simulink subsystem "Sensor"  (R2023b)
settings: Solver=VariableStepAuto  StartTime=0.0  StopTime=10.0  RelTol=1e-3
libraries: arduinosensorlib x2
settings Model: Creator=Usuario_UMA  LastModifiedBy=Diego

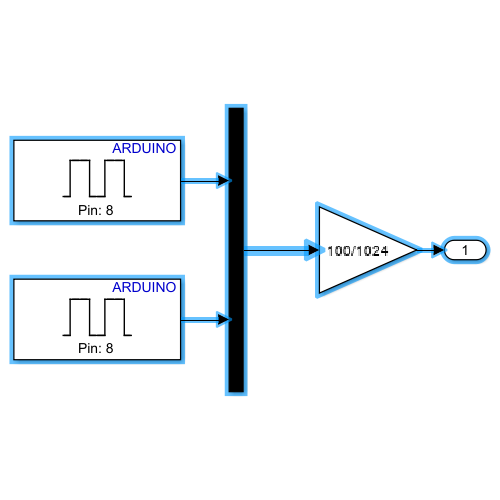
[thumbnail: Simulink's stored preview of the top-level diagram]
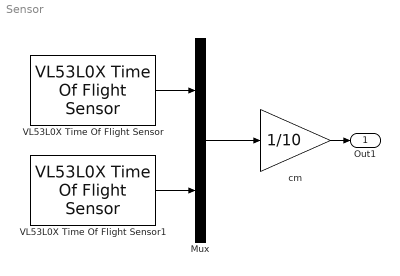
== system Sensor ==
  Mux : Mux  Inputs=2
  VL53L0X Time Of Flight Sensor : arduinosensorlib/VL53L0X Time Of Flight Sensor  I2CAddress=0x29  BitRate=1000000  RangingMode=Default  SampleTime=-1
  VL53L0X Time Of Flight Sensor1 : arduinosensorlib/VL53L0X Time Of Flight Sensor  I2CAddress=0x30  BitRate=1000000  RangingMode=Default  SampleTime=-1
  cm : Gain  Gain=1/10
  Out1 : Outport
  wires:
  cm/1 -> Out1/1
  VL53L0X Time Of Flight Sensor1/1 -> Mux/2
  VL53L0X Time Of Flight Sensor/1 -> Mux/1
  Mux/1 -> cm/1
